simulink model "testfun"  (R2015b)
settings: Solver=VariableStepAuto  StartTime=0.0  StopTime=10.0  RelTol=1e-3
values from neighbouring files (symbols this model uses):
  C = img(max(r2+(c1-1)*sx,1))    [IntegralImage_BoxIntegral_mine.m]
undefined symbols (not defined in the file or in its folder): gray, videoinput
libraries: imaqlib x1, visionsinks x1
settings Model: Creator=FLM  LastModifiedBy=FLM

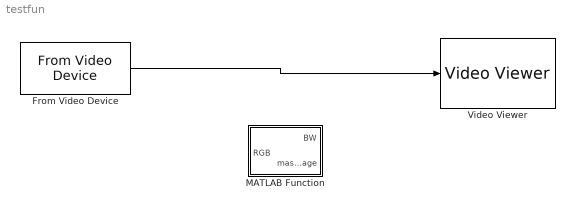
== system testfun ==
  From Video Device : imaqlib/From Video Device  DeviceMenu=winvideo 1 (Integrated Camera)  Device=winvideo 1 (Integrated Camera)  ObjConstructor=videoinput('winvideo', 1)  VideoFormatMenu=RGB24_640x480  VideoFormat=RGB24_640x480  VideoSource=input1  ROIPosition=[0 0 480 640]  EnableHWTrigger=off  TriggerConfiguration=winvideo 1 (Integrated Camera)  SampleTime=1/30  OutputPortsMode=One multidimensional signal  DataType=single  CanDoHWTrigger=no  ReturnedColorSpace=rgb  BlockHandle=1963.0012  ROIWidth=640  ROIHeight=480  ROIColumn=0  ROIRow=0  EngXMLPath=C:\Program Files\MATLAB\R2015b\toolbox\imaq\imaq\private  DevXMLPath=C:\MATLAB\SupportPackages\R2015b\osgenericvideointerface\toolbox\imaq\supportpackages\genericvideo\adaptor\win64  EngLibPath=C:\Program Files\MATLAB\R2015b\toolbox\imaq\imaqblks\imaqmex\win64  ColorSpace=rgb  BayerSensorAlignment=grbg
  MATLAB Function : MATLAB Function  TreatAsAtomicUnit=on
  Video Viewer : visionsinks/Video Viewer  inputType=Obsolete7b  imagePorts=One multidimensional signal  useColorMap=off  colormapValue=gray(256)  specRange=off  minInputVal=0  maxInputVal=255  FigPos=[854.6 805.2 409.6 300]  AxisZoom=on  trueSizedOnce=off  OpenAtMdlStart=on  DefaultConfigurationName=vipscopes.VideoViewerScopeCfg
  wires:
  From Video Device/1 -> Video Viewer/1

== matlab function testfun/MATLAB Function ==
  data: RGB input; BW output; maskedRGBImage output
function [BW,maskedRGBImage] = createMask_simu(RGB)
%createMask  Threshold RGB image using auto-generated code from colorThresholder app.
%  [BW,MASKEDRGBIMAGE] = createMask(RGB) thresholds image RGB using
%  auto-generated code from the colorThresholder App. The colorspace and
%  minimum/maximum values for each channel of the colorspace were set in the
%  App and result in a binary mask BW and a composite image maskedRGBImage,
%  which shows the original RGB image values under the mask BW.

% Auto-generated by colorThresholder app on 01-Mar-2016
%------------------------------------------------------


% Convert RGB image to chosen color space
I = rgb2hsv(RGB);

% Define thresholds for channel 1 based on histogram settings
channel1Min = 0.187;
channel1Max = 0.514;

% Define thresholds for channel 2 based on histogram settings
channel2Min = 0.196;
channel2Max = 1.000;

% Define thresholds for channel 3 based on histogram settings
channel3Min = 0.000;
channel3Max = 0.650;

% Create mask based on chosen histogram thresholds
BW = (I(:,:,1) >= channel1Min ) & (I(:,:,1) <= channel1Max) & ...
    (I(:,:,2) >= channel2Min ) & (I(:,:,2) <= channel2Max) & ...
    (I(:,:,3) >= channel3Min ) & (I(:,:,3) <= channel3Max);

% Initialize output masked image based on input image.
maskedRGBImage = RGB;

% Set background pixels where BW is false to zero.
maskedRGBImage(repmat(~BW,[1 1 3])) = 0;
